simulink model "Linear"  (R2021b)
settings: Solver=VariableStepAuto  StartTime=0.0  StopTime=100  RelTol=1e-3
undefined symbols (not defined in the file): A_numerical, B_numerical, C_numerical, D_numerical, inv_G_CL_0, K_d_LQR, K_q_LQR, K_statefeedback
settings Model: Creator=sadeg  LastModifiedBy=sadeg
settings SolverCC: AlgebraicLoopSolver=TrustRegion
settings SFSimCC: CustomCodeUndefinedFunction=UseInterfaceOnly

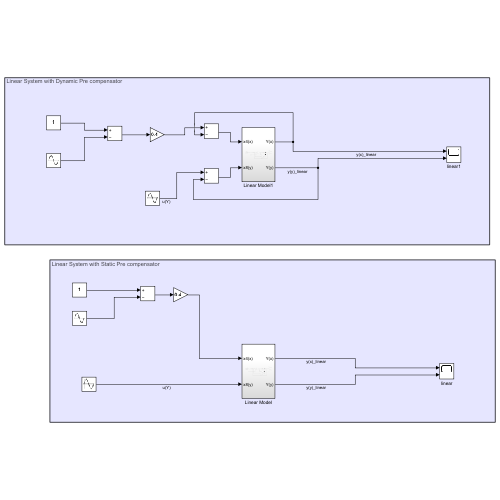
[thumbnail: Simulink's stored preview of the top-level diagram]
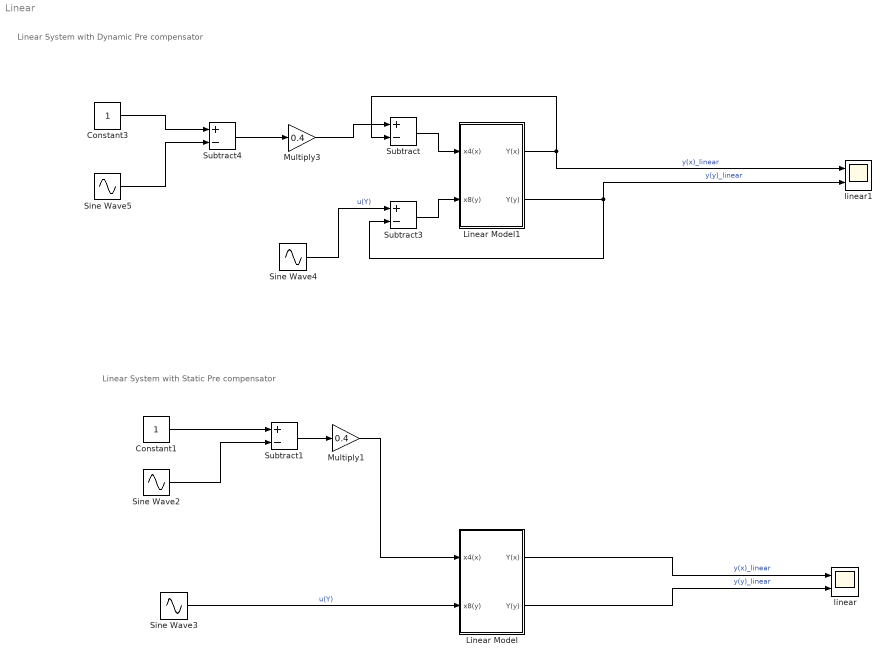
== system Linear ==
  note: Linear System with Static Pre compensator
  note: Linear System with Dynamic Pre compensator
  Constant1 : Constant
  Constant3 : Constant
  Linear Model : Subsystem
  Linear Model1 : Subsystem
  Multiply1 : Gain  Gain=0.4
  Multiply3 : Gain  Gain=0.4
  Sine Wave2 : Sin  Phase=pi/2  SampleTime=0
  Sine Wave3 : Sin  Amplitude=0.4  SampleTime=0
  Sine Wave4 : Sin  Amplitude=0.4  SampleTime=0
  Sine Wave5 : Sin  Phase=pi/2  SampleTime=0
  Subtract{,1,3..4} (4 alike) : Sum  Inputs=+-
  linear : Scope  NumInputPorts=2
  linear1 : Scope  NumInputPorts=2
  wires:
  Linear Model/1(Y(x)) -> linear/1  "y(x)_linear"
  Linear Model/2(Y(y)) -> linear/2  "y(y)_linear"
  Sine Wave3/1 -> Linear Model/2(x8(y))  "u(Y)"
  Subtract1/1 -> Multiply1/1
  Sine Wave2/1 -> Subtract1/2
  Constant1/1 -> Subtract1/1
  Multiply1/1 -> Linear Model/1(x4(x))
  Linear Model1/2(Y(y)) -> Subtract3/2, linear1/2  "y(y)_linear"
  Linear Model1/1(Y(x)) -> Subtract/2, linear1/1  "y(x)_linear"
  Subtract/1 -> Linear Model1/1(x4(x))
  Subtract3/1 -> Linear Model1/2(x8(y))
  Sine Wave5/1 -> Subtract4/2
  Subtract4/1 -> Multiply3/1
  Constant3/1 -> Subtract4/1
  Sine Wave4/1 -> Subtract3/1  "u(Y)"
  Multiply3/1 -> Subtract/1

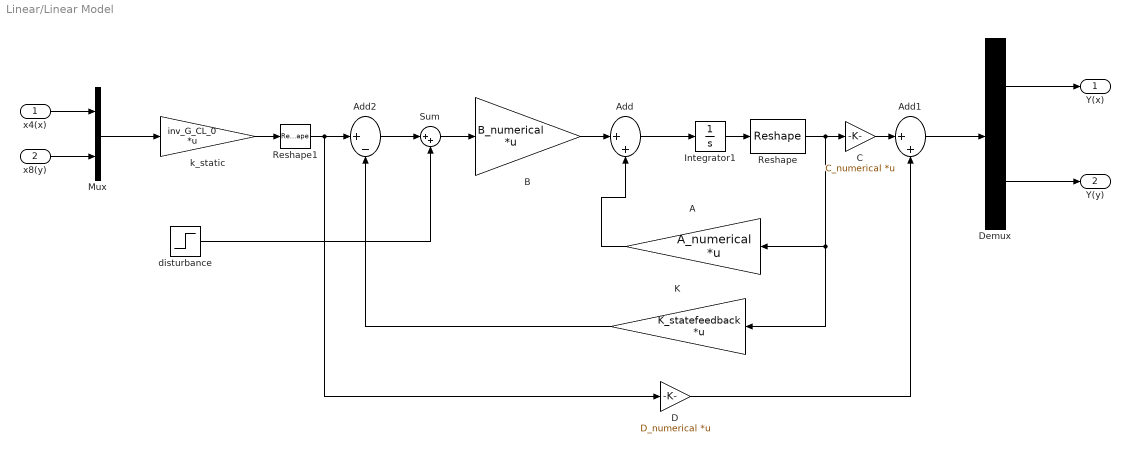
== system Linear/Linear Model ==
  x4(x) : Inport
  x8(y) : Inport  Port=2
  A : Gain  Gain=A_numerical  Multiplication=Matrix(K*u)
  Add : Sum  Inputs=|++
  Add1 : Sum  Inputs=|++
  Add2 : Sum  Inputs=|+-
  B : Gain  Gain=B_numerical  Multiplication=Matrix(K*u)
  C : Gain  Gain=C_numerical  Multiplication=Matrix(K*u)
  D : Gain  Gain=D_numerical  Multiplication=Matrix(K*u)
  Demux : Demux  Outputs=2
  Integrator1 : Integrator  InitialCondition=zeros(8,1)
  K : Gain  Gain=K_statefeedback  Multiplication=Matrix(K*u)
  Mux : Mux  Inputs=2
  Reshape : Reshape  OutputDimensionality=Column vector (2-D)
  Reshape1 : Reshape  OutputDimensionality=Column vector (2-D)
  Sum : Sum  Inputs=|++
  disturbance : Step  Time=3  After=0.5  SampleTime=0
  k_static : Gain  Gain=inv_G_CL_0  Multiplication=Matrix(K*u)
  Y(x) : Outport
  Y(y) : Outport  Port=2
  wires:
  Demux/2 -> Y(y)/1
  A/1 -> Add/2
  Integrator1/1 -> Reshape/1
  Reshape/1 -> A/1, K/1, C/1
  x4(x)/1 -> Mux/1
  C/1 -> Add1/1
  B/1 -> Add/1
  x8(y)/1 -> Mux/2
  Demux/1 -> Y(x)/1
  Add1/1 -> Demux/1
  Add/1 -> Integrator1/1
  D/1 -> Add1/2
  Reshape1/1 -> Add2/1, D/1
  K/1 -> Add2/2
  Mux/1 -> k_static/1
  k_static/1 -> Reshape1/1
  Add2/1 -> Sum/1
  Sum/1 -> B/1
  disturbance/1 -> Sum/2

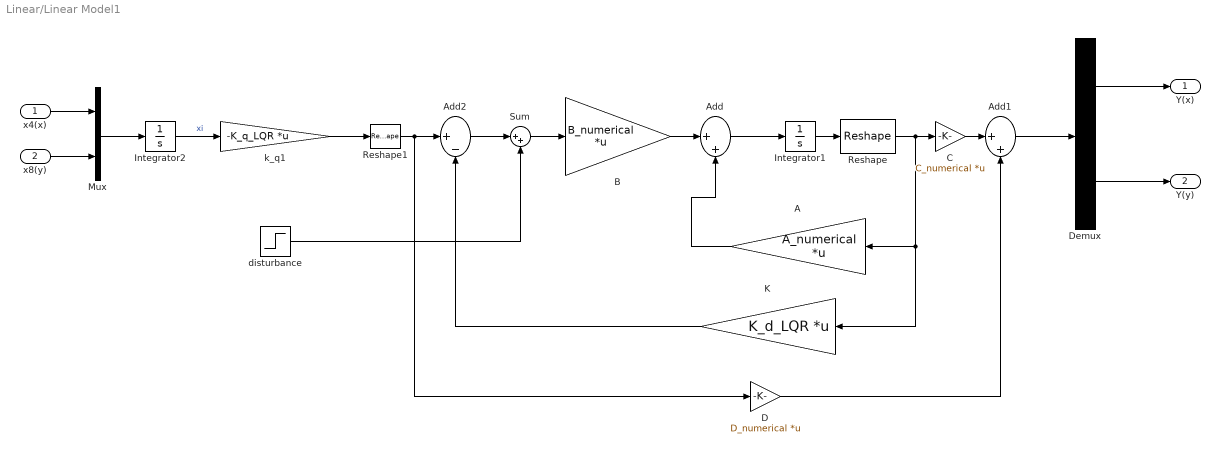
== system Linear/Linear Model1 ==
  x4(x) : Inport
  x8(y) : Inport  Port=2
  A : Gain  Gain=A_numerical  Multiplication=Matrix(K*u)
  Add : Sum  Inputs=|++
  Add1 : Sum  Inputs=|++
  Add2 : Sum  Inputs=|+-
  B : Gain  Gain=B_numerical  Multiplication=Matrix(K*u)
  C : Gain  Gain=C_numerical  Multiplication=Matrix(K*u)
  D : Gain  Gain=D_numerical  Multiplication=Matrix(K*u)
  Demux : Demux  Outputs=2
  Integrator1 : Integrator  InitialCondition=zeros(8,1)
  Integrator2 : Integrator
  K : Gain  Gain=K_d_LQR  Multiplication=Matrix(K*u)
  Mux : Mux  Inputs=2
  Reshape : Reshape  OutputDimensionality=Column vector (2-D)
  Reshape1 : Reshape  OutputDimensionality=Column vector (2-D)
  Sum : Sum  Inputs=|++
  disturbance : Step  Time=3  After=0.5  SampleTime=0
  k_q1 : Gain  Gain=-K_q_LQR  Multiplication=Matrix(K*u)
  Y(x) : Outport
  Y(y) : Outport  Port=2
  wires:
  Demux/2 -> Y(y)/1
  A/1 -> Add/2
  Integrator1/1 -> Reshape/1
  Reshape/1 -> A/1, K/1, C/1
  x4(x)/1 -> Mux/1
  C/1 -> Add1/1
  B/1 -> Add/1
  x8(y)/1 -> Mux/2
  Demux/1 -> Y(x)/1
  Add1/1 -> Demux/1
  Add/1 -> Integrator1/1
  D/1 -> Add1/2
  Reshape1/1 -> Add2/1, D/1
  K/1 -> Add2/2
  Mux/1 -> Integrator2/1
  k_q1/1 -> Reshape1/1
  Add2/1 -> Sum/1
  Sum/1 -> B/1
  disturbance/1 -> Sum/2
  Integrator2/1 -> k_q1/1  "xi"
